simulink model "filtro_dinamico_tracking"  (R2019a)
settings: Solver=VariableStepDiscrete  StartTime=0.0  StopTime=50  RelTol=1e-3  EnableMultiTasking=on
settings Model: Creator=david-herrera2  LastModifiedBy=PC-81597
settings DataIOCC: LimitDataPoints=on  SaveFormat=Array  ReturnWorkspaceOutputs=off
settings OptimizationCC: LifeSpan=inf
settings DebuggingCC: SolverPrmCheckMsg=warning  SFUnexpectedBacktrackingDiag=warning  SFNoUnconditionalDefaultTransitionDiag=warning  SFExecutionAtInitializationDiag=none  ArithmeticOperatorsInVariantConditions=warning
settings HardwareCC: ProdBitPerPointer=32  ProdBitPerSizeT=32  ProdBitPerPtrDiffT=32  ProdLargestAtomicFloat=None  ProdIntDivRoundTo=Undefined  ProdEndianess=Unspecified  ProdWordSize=32  ProdHWDeviceType=32-bit Generic
settings ModelReferenceCC: PropagateSignalLabelsOutOfModel=off
settings SFSimCC: SimUseLocalCustomCode=off
settings RTWCC: RTWUseLocalCustomCode=off
settings CodeAppCC: StateflowObjectComments=on
settings GRTTargetCC: TargetLangStandard=C89/C90 (ANSI)  GeneratePreprocessorConditionals=Disable all
settings ConfigComp: CovMetricSettings=dw  CovHtmlReporting=on  CovSaveCumulativeToWorkspaceVar=on  CovSaveSingleToWorkspaceVar=on  CovExternalEMLEnable=off  CovSFcnEnable=off

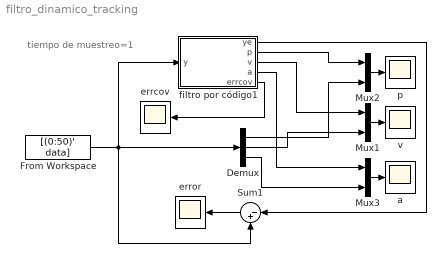
== system filtro_dinamico_tracking ==
  note: tiempo de muestreo=1
  " error" : Scope
  Demux : Demux  Outputs=3
  From Workspace : FromWorkspace  VariableName=[(0:50)' data]  SampleTime=1
  Mux1 : Mux  Inputs=2
  Mux2 : Mux  Inputs=2
  Mux3 : Mux  Inputs=2
  Sum1 : Sum  Inputs=|-+
  a : Scope
  errcov : Scope
  filtro por código1 : MATLAB Function  TreatAsAtomicUnit=on
  p : Scope
  v : Scope
  wires:
  From Workspace/1 -> filtro por código1/1(y), Demux/1, Sum1/2
  Mux2/1 -> p/1
  Sum1/1 -> " error"/1
  filtro por código1/5(errcov) -> errcov/1
  filtro por código1/1(ye) -> Sum1/1
  filtro por código1/2(p) -> Mux2/1
  Demux/1 -> Mux2/2
  Mux1/1 -> v/1
  filtro por código1/3(v) -> Mux1/1
  Demux/2 -> Mux1/2
  Mux3/1 -> a/1
  filtro por código1/4(a) -> Mux3/1
  Demux/3 -> Mux3/2

== matlab function filtro_dinamico_tracking/filtro por código1 ==
  data: ye output; y input; p output; v output; a output; errcov output
function [ye,p,v,a,errcov] = fcn(y)
%#codegen
Ts = 0.5;
F=[Ts*cos(0.2)*5 0 0;0 Ts*sin(0.2)*5 0;0 0 Ts*0.4]; 
H=eye(3);
persistent xe; % estados estimados, persistent para que lo mantenga en memoria
persistent P;
persistent K;
persistent R;
if isempty(xe)
        % R=diag(rand(3,1)); %aleatorio
        R=diag([225 16 0.04]); %del ejemplo
        xe = zeros(3,1);
end
if isempty(P)
        P=rand(3);
end

% esto debería ir en un ciclo infinito
% actualización en tiempo (predicción)
xe = F*xe;        % x[n+1|n]
P = F*P*F';     % P[n+1|n]

% actualización (medidas)
K = P*H'/(H*P*H'+R); % actualización de ganancia
xe = xe + K*(y-H*xe);  % x[n|n]
P = (eye(3)-K.*H)*P;  % P[n|n]

ye=H*xe; %salida estimada
p=ye(1);
v=ye(2);
a=ye(3);
errcov = H*P*H'; % actualización error covarianza
